simulink model "Skateboard_Suspension_Half_Board_Model_2_CTS_Simulink"  (R2022b)
settings: Solver=VariableStepAuto  StartTime=0.0  StopTime=10.0  RelTol=1e-3
values from neighbouring files (symbols this model uses):
  Cc = 0    [Skateboard_Suspension_Half_Board_Model_2_CTS.m]
  cF4 = (cbt*cbb)/(cbt + cbb)    [Skateboard_Suspension_Half_Board_Model_2_CTS.m]
  cw = 0    [Skateboard_Suspension_Half_Board_Model_2.m]    (also in Skateboard_Suspension_Half_Board_Model_2_CTS.m)
  kc = 0    [Skateboard_Suspension_Half_Board_Model_2_CTS.m]
  kF3 = (kbt*kbb)/(kbt + kbb)    [Skateboard_Suspension_Half_Board_Model_2_CTS.m]
  kw = 0    [Skateboard_Suspension_Half_Board_Model_2.m]    (also in Skateboard_Suspension_Half_Board_Model_2_CTS.m)
  mbt = 0    [Skateboard_Suspension_Half_Board_Model_2.m]    (also in Skateboard_Suspension_Half_Board_Model_2_CTS.m)
  mc = 0    [Skateboard_Suspension_Half_Board_Model_2_CTS.m]
  md = 0    [Skateboard_Suspension_Half_Board_Model_2.m]    (also in Skateboard_Suspension_Half_Board_Model_2_CTS.m)
  mtt = 0    [Skateboard_Suspension_Half_Board_Model_2.m]    (also in Skateboard_Suspension_Half_Board_Model_2_CTS.m)
settings Model: Creator=victo  LastModifiedBy=victo

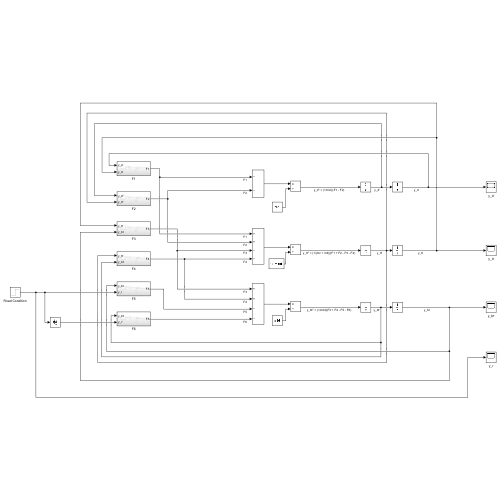
[thumbnail: Simulink's stored preview of the top-level diagram]
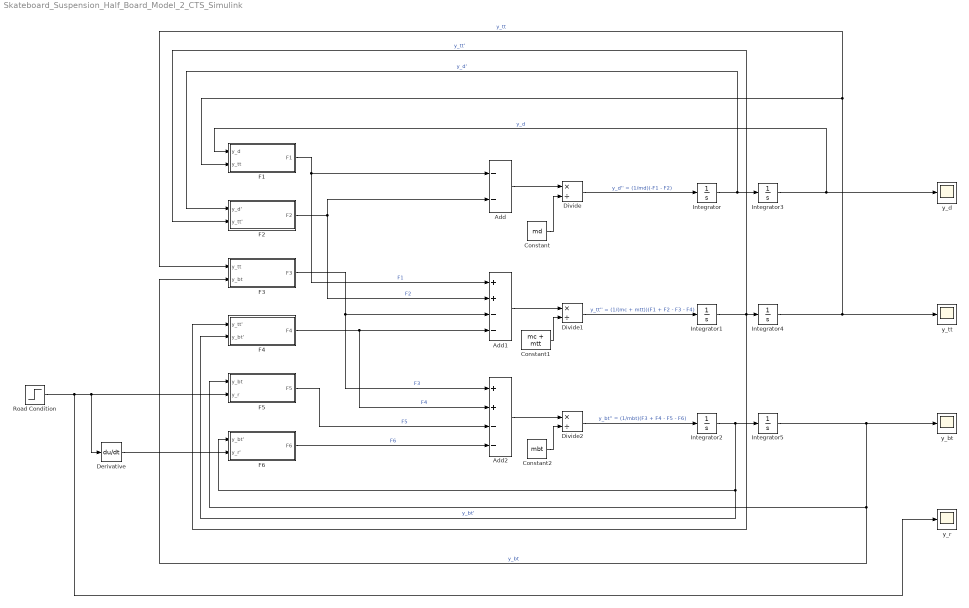
== system Skateboard_Suspension_Half_Board_Model_2_CTS_Simulink ==
  Add : Sum  Inputs=--
  Add1 : Sum  Inputs=++--
  Add2 : Sum  Inputs=++--
  Constant : Constant  Value=md
  Constant1 : Constant  Value=mc + mtt
  Constant2 : Constant  Value=mbt
  Derivative : Derivative
  Divide : Product  Inputs=*/
  Divide1 : Product  Inputs=*/
  Divide2 : Product  Inputs=*/
  F1 : Subsystem
  F2 : Subsystem
  F3 : Subsystem
  F4 : Subsystem
  F5 : Subsystem
  F6 : Subsystem
  Integrator{,1..5} (6 alike) : Integrator
  Road Condition : Step  SampleTime=0
  y_bt : Scope
  y_d : Scope
  y_r : Scope
  y_tt : Scope
  wires:
  Divide1/1 -> Integrator1/1  "y_tt'' = (1/(mc + mtt))(F1 + F2 - F3 - F4)"
  Integrator/1 -> Integrator3/1, F2/1(y_d')  "y_d'"
  Integrator2/1 -> F4/2(y_bt'), F6/1(y_bt'), Integrator5/1  "y_bt'"
  Integrator5/1 -> F3/2(y_bt), F5/1(y_bt), y_bt/1  "y_bt"
  Integrator3/1 -> y_d/1, F1/1(y_d)  "y_d"
  F1/1(F1) -> Add/1, Add1/1  "F1"
  F3/1(F3) -> Add2/1, Add1/3  "F3"
  Integrator1/1 -> F4/1(y_tt'), F2/2(y_tt'), Integrator4/1  "y_tt'"
  Derivative/1 -> F6/2(y_r')
  F4/1(F4) -> Add2/2, Add1/4  "F4"
  Integrator4/1 -> y_tt/1, F3/1(y_tt), F1/2(y_tt)  "y_tt"
  Divide2/1 -> Integrator2/1  "y_bt'' = (1/mbt)(F3 + F4 - F5 - F6)"
  Road Condition/1 -> y_r/1, Derivative/1, F5/2(y_r)
  F5/1(F5) -> Add2/3  "F5"
  F2/1(F2) -> Add/2, Add1/2  "F2"
  Divide/1 -> Integrator/1  "y_d'' = (1/md)(-F1 - F2)"
  Add2/1 -> Divide2/1
  F6/1(F6) -> Add2/4  "F6"
  Constant1/1 -> Divide1/2
  Constant/1 -> Divide/2
  Add1/1 -> Divide1/1
  Add/1 -> Divide/1
  Constant2/1 -> Divide2/2

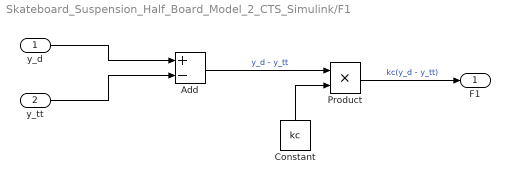
== system Skateboard_Suspension_Half_Board_Model_2_CTS_Simulink/F1 ==
  y_d : Inport
  y_tt : Inport  Port=2
  Add : Sum  Inputs=+-
  Constant : Constant  Value=kc
  Product : Product
  F1 : Outport
  wires:
  y_d/1 -> Add/1
  y_tt/1 -> Add/2
  Add/1 -> Product/1  "y_d - y_tt"
  Constant/1 -> Product/2
  Product/1 -> F1/1  "kc(y_d - y_tt)"

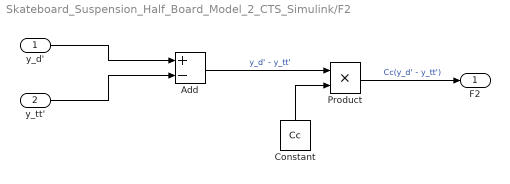
== system Skateboard_Suspension_Half_Board_Model_2_CTS_Simulink/F2 ==
  y_d' : Inport
  y_tt' : Inport  Port=2
  Add : Sum  Inputs=+-
  Constant : Constant  Value=Cc
  Product : Product
  F2 : Outport
  wires:
  y_d'/1 -> Add/1
  y_tt'/1 -> Add/2
  Add/1 -> Product/1  "y_d' - y_tt'"
  Constant/1 -> Product/2
  Product/1 -> F2/1  "Cc(y_d' - y_tt')"

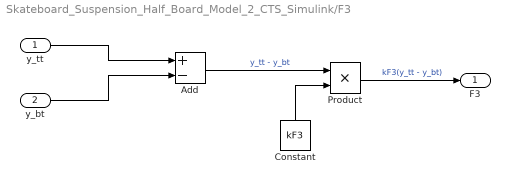
== system Skateboard_Suspension_Half_Board_Model_2_CTS_Simulink/F3 ==
  y_tt : Inport
  y_bt : Inport  Port=2
  Add : Sum  Inputs=+-
  Constant : Constant  Value=kF3
  Product : Product
  F3 : Outport
  wires:
  y_tt/1 -> Add/1
  y_bt/1 -> Add/2
  Add/1 -> Product/1  "y_tt - y_bt"
  Constant/1 -> Product/2
  Product/1 -> F3/1  "kF3(y_tt - y_bt)"

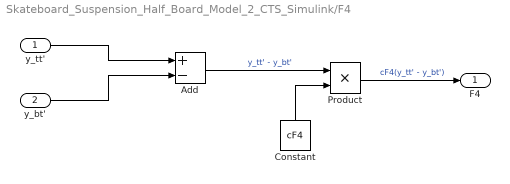
== system Skateboard_Suspension_Half_Board_Model_2_CTS_Simulink/F4 ==
  y_tt' : Inport
  y_bt' : Inport  Port=2
  Add : Sum  Inputs=+-
  Constant : Constant  Value=cF4
  Product : Product
  F4 : Outport
  wires:
  y_tt'/1 -> Add/1
  y_bt'/1 -> Add/2
  Add/1 -> Product/1  "y_tt' - y_bt'"
  Constant/1 -> Product/2
  Product/1 -> F4/1  "cF4(y_tt' - y_bt')"

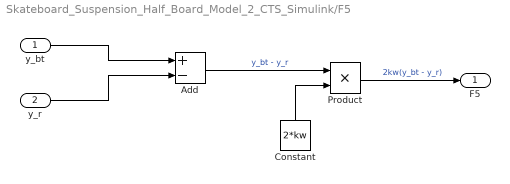
== system Skateboard_Suspension_Half_Board_Model_2_CTS_Simulink/F5 ==
  y_bt : Inport
  y_r : Inport  Port=2
  Add : Sum  Inputs=+-
  Constant : Constant  Value=2*kw
  Product : Product
  F5 : Outport
  wires:
  y_bt/1 -> Add/1
  y_r/1 -> Add/2
  Add/1 -> Product/1  "y_bt - y_r"
  Constant/1 -> Product/2
  Product/1 -> F5/1  "2kw(y_bt - y_r)"

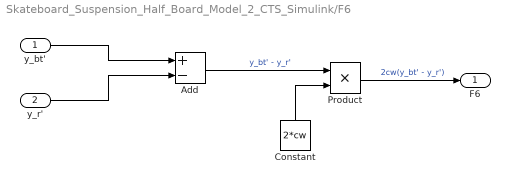
== system Skateboard_Suspension_Half_Board_Model_2_CTS_Simulink/F6 ==
  y_bt' : Inport
  y_r' : Inport  Port=2
  Add : Sum  Inputs=+-
  Constant : Constant  Value=2*cw
  Product : Product
  F6 : Outport
  wires:
  y_bt'/1 -> Add/1
  y_r'/1 -> Add/2
  Add/1 -> Product/1  "y_bt' - y_r'"
  Constant/1 -> Product/2
  Product/1 -> F6/1  "2cw(y_bt' - y_r')"
